simulink model "demo3e"  (Simulink 7.4)
settings: Solver=ode45  StartTime=0.0  StopTime=4  MaxStep=0.1  MinStep=0.01  RelTol=1e-3
undefined symbols (not defined in the file): observer, selectde, selectdx2e
libraries: roblocks x3, simulink x1
settings Model: Creator=pic  LastModifiedBy=acolome  ExtModeTrigMode=oneshot  ExtModeArmWhenConnect=off
settings DataIOCC: LimitDataPoints=off
settings OptimizationCC: BlockReduction=off  BooleanDataType=off  InitFltsAndDblsToZero=on
settings DebuggingCC: SaveWithParameterizedLinksMsg=none  SignalResolutionControl=TryResolveAllWithWarning  SolverPrmCheckMsg=none  MultiTaskDSMMsg=warning  MultiTaskCondExecSysMsg=none  StrictBusMsg=None
settings HardwareCC: TargetUnknown=on
settings RTWCC: IncludeERTFirstTime=on
settings GRTTargetCC: ModelReferenceCompliant=off  ParMdlRefBuildCompliant=off  CompOptLevelCompliant=off  MatFileLogging=off

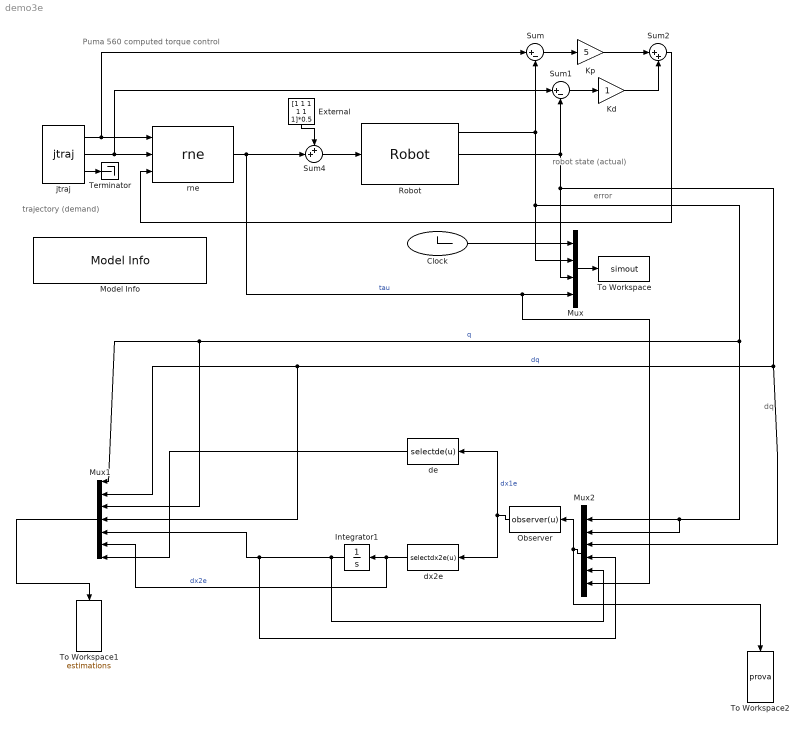
== system demo3e ==
  note: Puma 560 computed torque control
  note: trajectory
      | (demand)
  note: robot state
      | (actual)
  note: error
  note: dq
  Clock : Clock
      settings: Decimation=100
  External : Constant  Value=[1 1 1 1 1 1]*0.5  OutDataType=fixdt(1, 16)  OutScaling=2^0
  Integrator1 : Integrator  InitialCondition=[0 0 0 0 0 0]
  Kd : Gain  SaturateOnIntegerOverflow=on  OutDataTypeStr=Inherit: Same as input  ParamDataTypeStr=Inherit: Same as input
  Kp : Gain  Gain=5  SaturateOnIntegerOverflow=on  OutDataTypeStr=Inherit: Same as input  ParamDataTypeStr=Inherit: Same as input
  Model Info : simulink/Model-Wide Utilities/Model Info  SystemSampleTime=-1  InitialBlockCM=none  BlockCM=none  Frame=on  DisplayStringWithTags=|  HorizontalTextAlignment=Left  LeftAlignmentValue=0.02  SourceBlockDiagram=demo3e  TagMaxNumber=20
      | Puma560 computed torque control
      | %<Creator>
      | %<LastModificationDate>
  Mux : Mux
  Mux1 : Mux  Inputs=7
  Mux2 : Mux  Inputs=6
  Observer : MATLABFcn  MATLABFcn=observer(u)
  Robot : roblocks/Robot  SystemSampleTime=-1  robot=p560  q0=[0 0 0 0 0 0]
  Sum : Sum  Inputs=|+-  SaturateOnIntegerOverflow=on  InputSameDT=on  OutDataTypeStr=Inherit: Same as first input
  Sum1 : Sum  Inputs=|+-  SaturateOnIntegerOverflow=on  InputSameDT=on  OutDataTypeStr=Inherit: Same as first input
  Sum2 : Sum  Inputs=|++  SaturateOnIntegerOverflow=on  InputSameDT=on  OutDataTypeStr=Inherit: Same as first input
  Sum4 : Sum  Inputs=++|  OutDataType=fixdt(1, 16)  OutScaling=2^0
  Terminator : Terminator
  To Workspace : ToWorkspace  VariableName=simout  SampleTime=-1  SaveFormat=Array
  To Workspace1 : ToWorkspace  VariableName=estimations  SampleTime=-1  SaveFormat=Array
  To Workspace2 : ToWorkspace  VariableName=prova  SampleTime=-1  SaveFormat=Array
  de : MATLABFcn  MATLABFcn=selectde(u)
  dx2e : MATLABFcn  MATLABFcn=selectdx2e(u)
  jtraj : roblocks/jtraj  SystemSampleTime=-1  q0=[pi/4 pi/2 -pi/2 0 0 0]  qf=[pi/4 pi/2 -pi/2 0 0 0]  tmax=4
      link override MATLAB Fcn: MATLABFcn=squeeze(interp1(t,q,u))
      link override MATLAB Fcn1: MATLABFcn=squeeze(interp1(t,qd,u))
      link override MATLAB Fcn2: MATLABFcn=squeeze(interp1(t,qdd,u))
  rne : roblocks/rne  SystemSampleTime=-1  robot=p560  grav=[0 0 9.81]
  wires:
  Sum/1 -> Kp/1
  Kp/1 -> Sum2/1
  Robot/1 -> Sum/2, Mux/2, Mux1/1, Mux1/3, Mux2/1, Mux2/2  "q"
  Robot/2 -> Sum1/2, Mux/3, Mux2/3, Mux1/2, Mux1/4  "dq"
  Sum2/1 -> rne/3
  rne/1 -> Sum4/2, Mux/4, Mux2/6  "tau"
  jtraj/1 -> Sum/1, rne/1
  jtraj/2 -> rne/2, Sum1/1
  Mux/1 -> To Workspace/1
  Clock/1 -> Mux/1
  Sum1/1 -> Kd/1
  Kd/1 -> Sum2/2
  jtraj/3 -> Terminator/1
  Sum4/1 -> Robot/1
  External/1 -> Sum4/1
  Mux1/1 -> To Workspace1/1
  Mux2/1 -> Observer/1, To Workspace2/1
  Observer/1 -> de/1, dx2e/1  "dx1e"
  de/1 -> Mux1/7
  dx2e/1 -> Integrator1/1, Mux1/6  "dx2e"
  Integrator1/1 -> Mux2/5, Mux1/5, Mux2/4
